simulink model "Simulink_Scroll"  (Simulink 7.3)
settings: Solver=ode45  StartTime=0.0  StopTime=200  RelTol=1e-3
libraries: simulink_extras x3
settings Model: Creator=jocurrie  LastModifiedBy=Jonathan

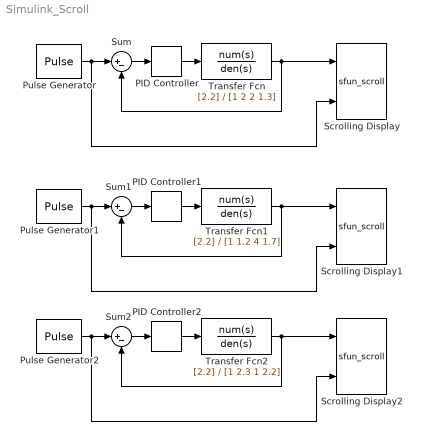
== system Simulink_Scroll ==
  PID Controller : simulink_extras/Additional Linear/PID Controller  SystemSampleTime=-1  P=0.3  I=0.3  D=0.3
  PID Controller1 : simulink_extras/Additional Linear/PID Controller  SystemSampleTime=-1  P=0.3  I=0.3  D=0.3
  PID Controller2 : simulink_extras/Additional Linear/PID Controller  SystemSampleTime=-1  P=0.1  I=0.1  D=0.1
  Pulse Generator : DiscretePulseGenerator  PulseType=Time based  Amplitude=10  Period=30  PulseWidth=50  PhaseDelay=0  SampleTime=1
  Pulse Generator1 : DiscretePulseGenerator  PulseType=Time based  Amplitude=0.1  Period=30  PulseWidth=50  PhaseDelay=0  SampleTime=1
  Pulse Generator2 : DiscretePulseGenerator  PulseType=Time based  Amplitude=1  Period=30  PulseWidth=50  PhaseDelay=0  SampleTime=1
  Scrolling Display : M-S-Function  FunctionName=sfun_scroll  Parameters=Ts,Frame_Size,Update_Delay,y_lim,setp  mask(Scrolling Plot){Ts=0.1, Frame_Size=200, Update_Delay=0.005, y_lim=[-1 1], setp=on}
      mask prompts: Ts "Sampling Time (Seconds)"; Frame_Size "Frame Size (Samples)"; Update_Delay "Update Delay (Seconds)"; y_lim "Initial Y axis Limits [ymin ymax]"; setp "Enable Set Point Input"
      mask help:
      | Create a scrolling, autoscaling display for use in Simulink
      |
      | The display is a discrete component, and requires a sampling period. Adjust this period for the desired resolution.
      |
      | Frame size refers to the number of samples to be displayed on the screen before it begins to scroll.
      |
      | Update delay allows a rough delay of the simulation execution period, allowing the user to slow down the display.
      mask init:
      | if(~Ts)
      |     disp('Warning: Sampling Time (Ts) Not Specifed or is Zero');
      |     Ts = 0.1;
      | end
      | 
      | if(~Frame_Size)
      |     disp('Warning: Frame Size Not Specifed or is Zero');
      |     Frame_Size = 100;
      | end
      | 
      | if(Update_Delay < 0)
      |     Update_Delay = 0;
      | else if(Update_Delay > 10)
      |         disp('Warning: Update Delay Specified as > 10'); 
      |         Update_Delay = 10;
      |     end
      | end
      | 
      | if(y_lim(1) > y_lim(2))
      |     disp('Warning: Limit 1 is greater than Limit 2');
      |     y_lim(1) = -y_lim(1);
      | end
      | if(y_lim(1) == y_lim(2))
      |     disp('Warning: Limits are equal');
      |     if(~y_lim(1))
      |         y_lim(2) = 1;
      |     else
      |         y_lim(2) = y_lim(2)+abs(y_lim(2));
      |     end
      | end
      mask Help: Note this block accepts a maximum of one input per port, if you connect a multiple dimsension signal results will be unpredictable.
      mask Display: image(imread('Scrollpic.jpg'))
  Scrolling Display1 : M-S-Function  FunctionName=sfun_scroll  Parameters=Ts,Frame_Size,Update_Delay,y_lim,setp  mask(Scrolling Plot){Ts=0.1, Frame_Size=200, Update_Delay=0, y_lim=[0 0.1], setp=on}
      mask prompts: Ts "Sampling Time (Seconds)"; Frame_Size "Frame Size (Samples)"; Update_Delay "Update Delay (Seconds)"; y_lim "Initial Y axis Limits [ymin ymax]"; setp "Enable Set Point Input"
      mask help:
      | Create a scrolling, autoscaling display for use in Simulink
      |
      | The display is a discrete component, and requires a sampling period. Adjust this period for the desired resolution.
      |
      | Frame size refers to the number of samples to be displayed on the screen before it begins to scroll.
      |
      | Update delay allows a rough delay of the simulation execution period, allowing the user to slow down the display.
      mask init: same as Simulink_Scroll/Scrolling Display
      mask Help: Note this block accepts a maximum of one input per port, if you connect a multiple dimsension signal results will be unpredictable.
      mask Display: image(imread('Scrollpic.jpg'))
  Scrolling Display2 : M-S-Function  FunctionName=sfun_scroll  Parameters=Ts,Frame_Size,Update_Delay,y_lim,setp  mask(Scrolling Plot){Ts=0.1, Frame_Size=200, Update_Delay=0, y_lim=[0 1], setp=on}
      mask prompts: Ts "Sampling Time (Seconds)"; Frame_Size "Frame Size (Samples)"; Update_Delay "Update Delay (Seconds)"; y_lim "Initial Y axis Limits [ymin ymax]"; setp "Enable Set Point Input"
      mask help:
      | Create a scrolling, autoscaling display for use in Simulink
      |
      | The display is a discrete component, and requires a sampling period. Adjust this period for the desired resolution.
      |
      | Frame size refers to the number of samples to be displayed on the screen before it begins to scroll.
      |
      | Update delay allows a rough delay of the simulation execution period, allowing the user to slow down the display.
      mask init: same as Simulink_Scroll/Scrolling Display
      mask Help: Note this block accepts a maximum of one input per port, if you connect a multiple dimsension signal results will be unpredictable.
      mask Display: image(imread('Scrollpic.jpg'))
  Sum : Sum  Inputs=|+-  OutDataType=fixdt(1, 16)  OutScaling=2^0
  Sum1 : Sum  Inputs=|+-  OutDataType=fixdt(1, 16)  OutScaling=2^0
  Sum2 : Sum  Inputs=|+-  OutDataType=fixdt(1, 16)  OutScaling=2^0
  Transfer Fcn : TransferFcn  Numerator=[2.2]  Denominator=[1 2 2 1.3]
  Transfer Fcn1 : TransferFcn  Numerator=[2.2]  Denominator=[1 1.2 4 1.7]
  Transfer Fcn2 : TransferFcn  Numerator=[2.2]  Denominator=[1 2.3 1 2.2]
  wires:
  Transfer Fcn/1 -> Sum/2, Scrolling Display/1
  Pulse Generator/1 -> Sum/1, Scrolling Display/2
  PID Controller/1 -> Transfer Fcn/1
  Sum/1 -> PID Controller/1
  Transfer Fcn1/1 -> Sum1/2, Scrolling Display1/1
  Pulse Generator1/1 -> Sum1/1, Scrolling Display1/2
  PID Controller1/1 -> Transfer Fcn1/1
  Sum1/1 -> PID Controller1/1
  Transfer Fcn2/1 -> Sum2/2, Scrolling Display2/1
  Pulse Generator2/1 -> Sum2/1, Scrolling Display2/2
  PID Controller2/1 -> Transfer Fcn2/1
  Sum2/1 -> PID Controller2/1
